simulink library "fft_library"  (Simulink 6.2)
values from neighbouring files (symbols this model uses):
  ActualCoeffs = exp(br_indices)    [butterfly_direct_mask.m]    (also in fft_stage_n_mask.m)
  MaxCoeffNum = 11    [biplex_core_mask.m]
  StepPeriod = FFTSize-FFTStage+max(0, FFTStage-MaxCoeffNum)    [fft_stage_n_mask.m]
  vlen = length(ActualCoeffs)    [fft_stage_n_mask.m]
undefined symbols (not defined in the file or in its folder): bit_reverse
libraries: xbsIndex_r3 x532, fft_library x29, delay_lib x9, reorder_library x7, twiddle_lib x1
(part 1 of 4)
settings Model: LastModifiedBy=hchen05

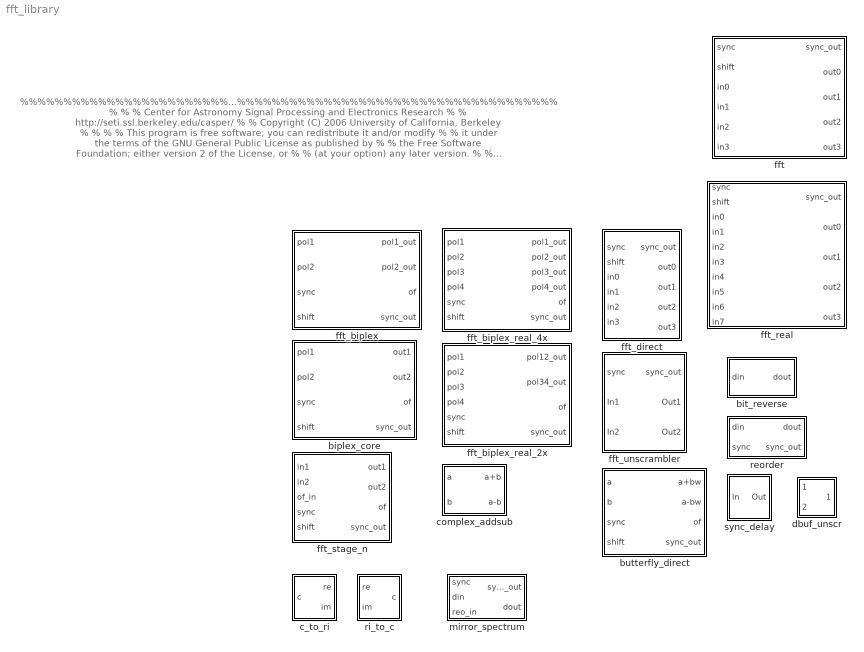
== system fft_library ==
  note: %%%%%%%%%%%%%%%%%%%%%%%%%%%%%%%%%%%%%%%%%%%%%%%%%%%%%%%%%%%%%%%%%%%%%%%%%%%%%%%
      | %                                                                             %
      | %   Center for Astronomy Signal Processing and Electronics Research           %
      | %   http://seti.ssl.berkeley.edu/casper/                                      %
      | %   Copyright (C) 2006 University of California, Berkeley                     %
      | %                                                                             %
      | %   This program is free software; you can redistribute it and/or modify      %
      | %   it under the terms of the GNU General Public License as published by      %
      | %   the Free Software Foundation; either version 2 of the License, or         %
      | %   (at your option) any later version.                                       %
      | %                                                                             %
      | %   This program is distributed in the hope that it will be useful,           %
      | %   but WITHOUT ANY WARRANTY; without even the implied warranty of            %
      | %   MERCHANTABILITY or FITNESS FOR A PARTICULAR PURPOSE.  See the             %
      | %   GNU General Public License for more details.                              %
      | %                                                                             %
      | %   You should have received a copy of the GNU General Public License along   %
      | %   with this program; if not, write to the Free Software Foundation, Inc.,   %
      | %   51 Franklin Street, Fifth Floor, Boston, MA 02110-1301 USA.               %
      | %                                                                             %
      | %%%%%%%%%%%%%%%%%%%%%%%%%%%%%%%%%%%%%%%%%%%%%%%%%%%%%%%%%%%%%%%%%%%%%%%%%%%%%%%
  biplex_core : Subsystem  mask{FFTSize=2, BitWidth=18, quantization=Truncate, overflow=Wrap, add_latency=2, mult_latency=3, bram_latency=2}
      mask prompts: FFTSize "Size of FFT: (2^? pnts)"; BitWidth "Bitwidth: (Max Efficiency at 18 bits)"; quantization "Quantization Behavior"; overflow "Overflow Behavior"; add_latency "Add Latency"; mult_latency "Mult Latency"; bram_latency "BRAM Latency"
      mask init:
      | biplex_core_mask;
      mask StyleString: edit,edit,popup(Truncate|Round  (unbiased: +/- Inf)|Round  (unbiased: Even Values)),popup(Wrap|Saturate|Error),edit,edit,edit
  bit_reverse : Subsystem  mask{n_bits=3}
      mask prompts: n_bits "Number of bits"
      mask init:
      | bit_reverse_mask;
      mask Display: fprintf('%d bits', n_bits)
  butterfly_direct : Subsystem  mask(butterfly_direct){FFTSize=5, Coeffs=0:3, StepPeriod=0, BitWidth=18, add_latency=4, mult_latency=4, bram_latency=4, use_bram=off, quantization=Round  (unbiased: Even Values), overflow=Wrap}
      mask prompts: FFTSize "Size of FFT: (2^?)"; Coeffs "Coefficients: (0 to 2^(FFTSize-1)-1)"; StepPeriod "Coefficient Step Period: (2^?)"; BitWidth "Output Bitwidth:"; add_latency "Add Latency"; mult_latency "Mult Latency"; bram_latency "BRAM Latency"; use_bram "Store Coefficients in BRAM"; quantization "Quantization Behavior"; overflow "Overflow Behavior"
      mask init:
      | butterfly_direct_mask;
      mask StyleString: edit,edit,edit,edit,edit,edit,edit,checkbox,popup(Truncate|Round  (unbiased: +/- Inf)|Round  (unbiased: Even Values)),popup(Wrap|Saturate|Error)
  c_to_ri : Subsystem  mask{BitWidth=18}
      mask prompts: BitWidth "Bit Width:"
  complex_addsub : Subsystem  mask{BitWidth=18, add_latency=2}
      mask prompts: BitWidth "Bit Wdith?"; add_latency "add latency?"
  dbuf_unscr : Subsystem  mask(dbuf_unscr){FFTSize=5, n_inputs=2, banknum=1, bram_latency=4}
      mask prompts: FFTSize "Size of FFT: (2^?)"; n_inputs "Number of Simultaneous Inputs: (2^?)"; banknum "Handling input #: (1 to # inputs)"; bram_latency "BRAM Latency"
      mask init:
      | biplex_len = FFTSize - n_inputs;
      | r = biplex_len - n_inputs;
  fft : Subsystem  mask{FFTSize=5, BitWidth=18, n_inputs=2, quantization=Round  (unbiased: Even Values), overflow=Wrap, add_latency=2, mult_latency=3, bram_latency=2}
      mask prompts: FFTSize "Size of FFT: (2^?)"; BitWidth "Bit Width"; n_inputs "Number of Simultaneous Inputs: (2^?)"; quantization "Quantization Behavior"; overflow "Overflow Behavior"; add_latency "Add Latency"; mult_latency "Mult Latency"; bram_latency "BRAM Latency"
      mask init:
      | fft_mask;
      mask StyleString: edit,edit,edit,popup(Truncate|Round  (unbiased: +/- Inf)|Round  (unbiased: Even Values)),popup(Wrap|Saturate|Error),edit,edit,edit
  fft_biplex : Subsystem  mask(fft_biplex){FFTSize=2, BitWidth=18, quantization=Truncate, overflow=Wrap, add_latency=2, mult_latency=3, bram_latency=2}
      mask prompts: FFTSize "Size of FFT: (2^? pnts)"; BitWidth "Bitwidth: (Max Efficiency at 18 bits)"; quantization "Quantization Behavior"; overflow "Overflow Behavior"; add_latency "Add Latency"; mult_latency "Mult Latency"; bram_latency "BRAM Latency"
      mask init:
      | cursys = gcb;
      | disp(cursys);
      | biplex_core = [cursys,'/biplex_core'];
      | if ~strcmp(get_param(biplex_core, 'quantization'), quantization),
      |     set_param(biplex_core, 'quantization', quantization);
      | end
      | if ~strcmp(get_param(biplex_core, 'overflow'), overflow),
      |     set_param(biplex_core, 'overflow', overflow);
      | end
      mask StyleString: edit,edit,popup(Truncate|Round  (unbiased: +/- Inf)|Round  (unbiased: Even Values)),popup(Wrap|Saturate|Error),edit,edit,edit
  fft_biplex_real_2x : Subsystem  mask{FFTSize=2, BitWidth=18, quantization=Round  (unbiased: Even Values), overflow=Wrap, add_latency=2, mult_latency=3, bram_latency=2}
      mask prompts: FFTSize "Size of FFT: (2^? pnts)"; BitWidth "Bitwidth: (Max Efficiency at 18 bits)"; quantization "Quantization Behavior"; overflow "Overflow Behavior"; add_latency "Add Latency"; mult_latency "Mult Latency"; bram_latency "BRAM Latency"
      mask init:
      | cursys = gcb;
      | disp(cursys);
      | biplex_core = [cursys,'/biplex_core'];
      | if ~strcmp(get_param(biplex_core, 'quantization'), quantization),
      |     set_param(biplex_core, 'quantization', quantization);
      | end
      mask StyleString: edit,edit,popup(Truncate|Round  (unbiased: +/- Inf)|Round  (unbiased: Even Values)),popup(Wrap|Saturate|Error),edit,edit,edit
  fft_biplex_real_4x : Subsystem  mask(fft_biplex_real_4x){FFTSize=4, BitWidth=18, quantization=Round  (unbiased: Even Values), overflow=Wrap, add_latency=2, mult_latency=3, bram_latency=2}
      mask prompts: FFTSize "Size of FFT: (2^? pnts)"; BitWidth "Bitwidth: (Max Efficiency at 18 bits)"; quantization "Quantization Behavior"; overflow "Overflow Behavior"; add_latency "Add Latency"; mult_latency "Mult Latency"; bram_latency "BRAM Latency"
      mask init:
      | cursys = gcb;
      | disp(cursys);
      | 
      | BRAMSize = 18432;
      | DelayBramThresh = 1/4;  % Use bram when delays will fill this fraction of a BRAM
      | 
      | biplex_core = [cursys,'/biplex_core'];
      | if ~strcmp(get_param(biplex_core, 'quantization'), quantization),
      |     set_param(biplex_core, 'quantization', quantization);
      | end
      | 
      | % Implement delays normally or in BRAM
      | 
      | if (2^(FFTSize-1) * 2*BitWidth >= DelayBramThresh*BRAMSize),
      |     delay_bram = 'on';
      | else,
      |     delay_bram = 'off';
      | end
      | 
      | delays = {'delay0', 'delay1'};
      | for i=1:length(delays),
      |     full_path = [cursys,'/bi_real_unscr_4x/',delays{i}];
      |     if 2^(FFTSize-1) > 16,
      |         delay_type = 'delay_bram';
      |     else,
      |         delay_type = 'delay_slr';
      |     end
      |     if ~strcmp(get_param(full_path, 'BlockChoice'), delay_type),
      |         set_param(full_path, 'BlockChoice', delay_type)
      |     end
      | end
      mask StyleString: edit,edit,popup(Truncate|Round  (unbiased: +/- Inf)|Round  (unbiased: Even Values)),popup(Wrap|Saturate|Error),edit,edit,edit
  fft_direct : Subsystem  mask{FFTSize=2, BitWidth=18, add_latency=2, mult_latency=3, bram_latency=2, quantization=Truncate, overflow=Wrap, MapTail=off, LargerFFTSize=5, StartStage=3}
      mask prompts: FFTSize "Size of FFT: (2^?)"; BitWidth "Bit Width"; add_latency "Add Latency"; mult_latency "Mult Latency"; bram_latency "BRAM Latency"; quantization "Quantization Behavior"; overflow "Overflow Behavior"; MapTail "Map Tail of Larger FFT"; LargerFFTSize "Size of Larger FFT (2^?):"; StartStage "Start Stage of Map Tail:"
      mask init:
      | fft_direct_mask;
      mask StyleString: edit,edit,edit,edit,edit,popup(Truncate|Round  (unbiased: +/- Inf)|Round  (unbiased: Even Values)),popup(Wrap|Saturate|Error),checkbox,edit,edit
      mask CallbackString:
      | |||||||if strcmp(get_param(gcb,'Maptail'),'on')
      |     set_param(gcb,'MaskVisibilities',{'on','on','on','on','on','on','on','on','on','on'});
      | else
      |     set_param(gcb,'MaskVisibilities',{'on','on','on','on','on','on','on','on','off','off'});
      | end||
  fft_real : Subsystem  mask{FFTSize=8, BitWidth=18, n_inputs=3, quantization=Round  (unbiased: Even Values), overflow=Wrap, add_latency=2, mult_latency=3, bram_latency=2}
      mask prompts: FFTSize "Size of FFT: (2^?)"; BitWidth "Bit Width"; n_inputs "Number of Simultaneous Inputs: (2^?)"; quantization "Quantization Behavior"; overflow "Overflow Behavior"; add_latency "Add Latency"; mult_latency "Mult Latency"; bram_latency "BRAM Latency"
      mask init:
      | fft_real_mask;
      mask StyleString: edit,edit,edit,popup(Truncate|Round  (unbiased: +/- Inf)|Round  (unbiased: Even Values)),popup(Wrap|Saturate|Error),edit,edit,edit
  fft_stage_n : Subsystem  mask(fft_stage){FFTSize=5, FFTStage=3, BitWidth=18, DelayBram=off, CoeffBram=off, MaxCoeffNum=12, quantization=Truncate, overflow=Wrap, add_latency=3, mult_latency=2, bram_latency=2}
      mask prompts: FFTSize "Size of FFT: (2^? pnts)"; FFTStage "Stage of FFT:"; BitWidth "Output Bitwidth:"; DelayBram "Implement Delays in BRAM:"; CoeffBram "Store Coefficients in BRAM:"; MaxCoeffNum "Maximum Coefficient Depth: (2^?)"; quantization "Quantization Behavior"; overflow "Overflow Behavior"; add_latency "Add Latency"; mult_latency "Mult Latency"; bram_latency "BRAM Latency"
      mask init:
      | fft_stage_n_mask;
      mask StyleString: edit,edit,edit,checkbox,checkbox,edit,popup(Truncate|Round  (unbiased: +/- Inf)|Round  (unbiased: Even Values)),popup(Wrap|Saturate|Error),edit,edit,edit
  fft_unscrambler : Subsystem  mask{FFTSize=6, n_inputs=1, bram_latency=2}
      mask prompts: FFTSize "Size of FFT: (2^?)"; n_inputs "Number of Simultaneous Inputs: (2^?)"; bram_latency "BRAM Latency"
      mask init:
      | fft_unscrambler_mask;
  mirror_spectrum : Subsystem  mask{FFTSize=4, n_bits=18, reorder_latency=2}
      mask prompts: FFTSize "FFT Size (2^?):"; n_bits "Bit Width"; reorder_latency "Reorder Latency"
  reorder : Subsystem  mask{n_bits=2, bit_reverse=off, ping_pong=off, bram_latency=2}
      mask prompts: n_bits "Length of Vector: (2^?)"; bit_reverse "Bit Reverse"; ping_pong "Backwards"; bram_latency "BRAM Latency"
      mask init:
      | cursys = gcb;
      | disp(cursys);
      | set_param([cursys,'/crazy_cnt'], 'bit_reverse', bit_reverse);
      | set_param([cursys,'/crazy_cnt'], 'ping_pong', ping_pong);
  ri_to_c : Subsystem  mask{likes_cookies=off}
      mask prompts: likes_cookies "I think cookies are delicious"
  sync_delay : Subsystem  mask{DelayLen=4}
      mask prompts: DelayLen "Delay Length:"
      mask init:
      | BitWidth = max(2, ceil(log2(DelayLen+1)));
      | UseCounter = 1;
      | if DelayLen == 0,
      | 	UseCounter = 0;
      | end
      mask Display: fprintf('Z^-%d', DelayLen)

== system fft_library/biplex_core ==
  pol1 : Inport  Port=1  LatchInput=off
  pol2 : Inport  Port=2  LatchInput=off
  sync : Inport  Port=3  LatchInput=off
  shift : Inport  Port=4  LatchInput=off
  fft_stage_1 : Subsystem  mask(fft_stage){FFTSize=FFTSize, FFTStage=1, BitWidth=BitWidth, DelayBram=off, CoeffBram=off, MaxCoeffNum=MaxCoeffNum, quantization=Truncate, overflow=Wrap, add_latency=add_latency, mult_latency=mult_latency, bram_latency=bram_latency}
      mask prompts: FFTSize "Size of FFT: (2^? pnts)"; FFTStage "Stage of FFT:"; BitWidth "Output Bitwidth:"; DelayBram "Implement Delays in BRAM:"; CoeffBram "Store Coefficients in BRAM:"; MaxCoeffNum "Maximum Coefficient Depth: (2^?)"; quantization "Quantization Behavior"; overflow "Overflow Behavior"; add_latency "Add Latency"; mult_latency "Mult Latency"; bram_latency "BRAM Latency"
      mask init:
      | fft_stage_n_mask;
      mask StyleString: edit,edit,edit,checkbox,checkbox,edit,popup(Truncate|Round  (unbiased: +/- Inf)|Round  (unbiased: Even Values)),popup(Wrap|Saturate|Error),edit,edit,edit
  fft_stage_2 : Subsystem  mask(fft_stage){FFTSize=FFTSize, FFTStage=2, BitWidth=BitWidth, DelayBram=off, CoeffBram=off, MaxCoeffNum=MaxCoeffNum, quantization=Truncate, overflow=Wrap, add_latency=add_latency, mult_latency=mult_latency, bram_latency=bram_latency}
      mask prompts: FFTSize "Size of FFT: (2^? pnts)"; FFTStage "Stage of FFT:"; BitWidth "Output Bitwidth:"; DelayBram "Implement Delays in BRAM:"; CoeffBram "Store Coefficients in BRAM:"; MaxCoeffNum "Maximum Coefficient Depth: (2^?)"; quantization "Quantization Behavior"; overflow "Overflow Behavior"; add_latency "Add Latency"; mult_latency "Mult Latency"; bram_latency "BRAM Latency"
      mask init:
      | fft_stage_n_mask;
      mask StyleString: edit,edit,edit,checkbox,checkbox,edit,popup(Truncate|Round  (unbiased: +/- Inf)|Round  (unbiased: Even Values)),popup(Wrap|Saturate|Error),edit,edit,edit
  out1 : Outport
  out2 : Outport  Port=2
  of : Outport  Port=3
  sync_out : Outport  Port=4
  wires:
  pol1/1 -> fft_stage_1/1(in1)
  pol2/1 -> fft_stage_1/2(in2)
  sync/1 -> fft_stage_1/3(sync)
  shift/1 -> fft_stage_1/4(shift), fft_stage_2/5(shift)
  fft_stage_1/1(out1) -> fft_stage_2/1(in1)
  fft_stage_1/2(out2) -> fft_stage_2/2(in2)
  fft_stage_1/3(of) -> fft_stage_2/3(of_in)
  fft_stage_1/4(sync_out) -> fft_stage_2/4(sync)
  fft_stage_2/1(out1) -> out1/1
  fft_stage_2/2(out2) -> out2/1
  fft_stage_2/3(of) -> of/1
  fft_stage_2/4(sync_out) -> sync_out/1

== system fft_library/bit_reverse ==
  din : Inport  Port=1  LatchInput=off
  Concat : xbsIndex_r3/Concat  num_inputs=3  explicit_period=off  period=1  dbl_ovrd=off
  slice0 : xbsIndex_r3/Slice  mode=Lower Bit Location + Width  nbits=1  bit1=0  base1=MSB of Input  bit0=0  base0=LSB of Input  boolean_output=off  explicit_period=off  period=1  dbl_ovrd=off
  slice1 : xbsIndex_r3/Slice  mode=Lower Bit Location + Width  nbits=1  bit1=0  base1=MSB of Input  bit0=1  base0=LSB of Input  boolean_output=off  explicit_period=off  period=1  dbl_ovrd=off
  slice2 : xbsIndex_r3/Slice  mode=Lower Bit Location + Width  nbits=1  bit1=0  base1=MSB of Input  bit0=2  base0=LSB of Input  boolean_output=off  explicit_period=off  period=1  dbl_ovrd=off
  dout : Outport
  wires:
  din/1 -> slice0/1, slice1/1, slice2/1
  slice0/1 -> Concat/1
  slice1/1 -> Concat/2
  slice2/1 -> Concat/3
  Concat/1 -> dout/1

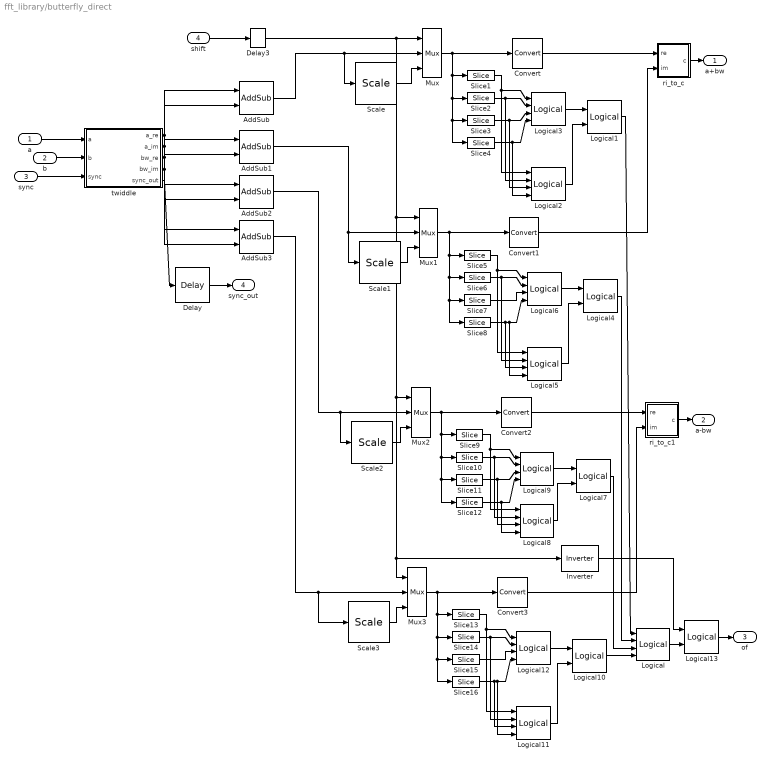
== system fft_library/butterfly_direct ==
  a : Inport  Port=1  LatchInput=off
  b : Inport  Port=2  LatchInput=off
  sync : Inport  Port=3  LatchInput=off
  shift : Inport  Port=4  LatchInput=off
  AddSub : xbsIndex_r3/AddSub  mode=Addition  precision=Full  arith_type=Unsigned  n_bits=8  bin_pt=2  quantization=Truncate  overflow=Wrap  latency=add_latency  explicit_period=off  period=1  use_carryin=off  use_carryout=off  en=off  dbl_ovrd=off  show_param=on  use_core=on  pipeline=on  use_rpm=on  gen_core=on
      settings: xl_area=[0, 0, 0, 0, 0, 0, 0]
  AddSub1 : xbsIndex_r3/AddSub  mode=Addition  precision=Full  arith_type=Unsigned  n_bits=8  bin_pt=2  quantization=Truncate  overflow=Wrap  latency=add_latency  explicit_period=off  period=1  use_carryin=off  use_carryout=off  en=off  dbl_ovrd=off  show_param=on  use_core=on  pipeline=on  use_rpm=on  gen_core=on
      settings: xl_area=[0, 0, 0, 0, 0, 0, 0]
  AddSub2 : xbsIndex_r3/AddSub  mode=Subtraction  precision=Full  arith_type=Unsigned  n_bits=8  bin_pt=2  quantization=Truncate  overflow=Wrap  latency=add_latency  explicit_period=off  period=1  use_carryin=off  use_carryout=off  en=off  dbl_ovrd=off  show_param=on  use_core=on  pipeline=on  use_rpm=on  gen_core=on
      settings: xl_area=[0, 0, 0, 0, 0, 0, 0]
  AddSub3 : xbsIndex_r3/AddSub  mode=Subtraction  precision=Full  arith_type=Unsigned  n_bits=8  bin_pt=2  quantization=Truncate  overflow=Wrap  latency=add_latency  explicit_period=off  period=1  use_carryin=off  use_carryout=off  en=off  dbl_ovrd=off  show_param=on  use_core=on  pipeline=on  use_rpm=on  gen_core=on
      settings: xl_area=[0, 0, 0, 0, 0, 0, 0]
  Convert{,1..3} (4 alike) : xbsIndex_r3/Convert  arith_type="Signed  (2's comp)"  n_bits=BitWidth  bin_pt=BitWidth-1  quantization="Round  (unbiased: Even Values)"  overflow=Wrap  latency=add_latency  explicit_period=off  period=1  dbl_ovrd=off  show_param=off  inserted_by_tool=off  pipeline=off
      settings: xl_area=[0, 0, 0, 0, 0, 0, 0]
  Delay : xbsIndex_r3/Delay  latency=2 * add_latency + 1  reg_retiming=off  explicit_period=off  period=1  en=off  accept_only_valid=off  init_zero=on  dbl_ovrd=off  show_param=off
      settings: xl_area=[0, 0, 0, 0, 0, 0, 0]
  Delay3 : xbsIndex_r3/Delay  latency=1  reg_retiming=off  explicit_period=off  period=1  en=off  accept_only_valid=off  init_zero=on  dbl_ovrd=off  show_param=off
      settings: xl_area=[0, 0, 0, 0, 0, 0, 0]
  Inverter : xbsIndex_r3/Inverter  latency=0  explicit_period=off  period=1  en=off  dbl_ovrd=off  show_param=off
      settings: xl_area=[0, 0, 0, 0, 0, 0, 0]
  Logical : xbsIndex_r3/Logical  logical_function=OR  inputs=4  precision=Full  arith_type=Unsigned  n_bits=8  bin_pt=2  align_bp=on  latency=1  explicit_period=off  period=1  en=off  dbl_ovrd=off  show_param=off
      settings: xl_area=[0, 0, 0, 0, 0, 0, 0]
  Logical{1,4,7,10} (4 alike) : xbsIndex_r3/Logical  logical_function=OR  inputs=2  precision=Full  arith_type=Unsigned  n_bits=8  bin_pt=2  align_bp=off  latency=1  explicit_period=off  period=1  en=off  dbl_ovrd=off  show_param=off
      settings: xl_area=[0, 0, 0, 0, 0, 0, 0]
  Logical{2,5,8,11} (4 alike) : xbsIndex_r3/Logical  logical_function=NOR  inputs=4  precision=Full  arith_type=Unsigned  n_bits=8  bin_pt=2  align_bp=off  latency=1  explicit_period=off  period=1  en=off  dbl_ovrd=off  show_param=off
      settings: xl_area=[0, 0, 0, 0, 0, 0, 0]
  Logical{3,6,9,12} (4 alike) : xbsIndex_r3/Logical  logical_function=AND  inputs=4  precision=Full  arith_type=Unsigned  n_bits=8  bin_pt=2  align_bp=off  latency=1  explicit_period=off  period=1  en=off  dbl_ovrd=off  show_param=off
      settings: xl_area=[0, 0, 0, 0, 0, 0, 0]
  Logical13 : xbsIndex_r3/Logical  logical_function=AND  inputs=2  precision=Full  arith_type=Unsigned  n_bits=8  bin_pt=2  align_bp=off  latency=1  explicit_period=off  period=1  en=off  dbl_ovrd=off  show_param=off
      settings: xl_area=[0, 0, 0, 0, 0, 0, 0]
  Mux{,1..3} (4 alike) : xbsIndex_r3/Mux  inputs=2  precision=Full  arith_type="Signed  (2's comp)"  n_bits=8  bin_pt=2  quantization=Truncate  overflow=Wrap  latency=1  explicit_period=off  period=1  en=off  dbl_ovrd=off  show_param=off  mux_type=off  use_rpm=off  gen_core=off
      settings: xl_area=[0, 0, 0, 0, 0, 0, 0]
  Scale{,1..3} (4 alike) : xbsIndex_r3/Scale  scale_factor=-1  explicit_period=off  period=1  dbl_ovrd=off
  Slice{1,5,9,13} (4 alike) : xbsIndex_r3/Slice  mode=Upper Bit Location + Width  nbits=1  bit1=0  base1=MSB of Input  bit0=0  base0=LSB of Input  boolean_output=on  explicit_period=off  period=1  dbl_ovrd=off
  Slice{2,6,10,14} (4 alike) : xbsIndex_r3/Slice  mode=Upper Bit Location + Width  nbits=1  bit1=-1  base1=MSB of Input  bit0=0  base0=LSB of Input  boolean_output=on  explicit_period=off  period=1  dbl_ovrd=off
  Slice{3,7,11,15} (4 alike) : xbsIndex_r3/Slice  mode=Upper Bit Location + Width  nbits=1  bit1=-2  base1=MSB of Input  bit0=0  base0=LSB of Input  boolean_output=on  explicit_period=off  period=1  dbl_ovrd=off
  Slice{4,8,12,16} (4 alike) : xbsIndex_r3/Slice  mode=Upper Bit Location + Width  nbits=1  bit1=-3  base1=MSB of Input  bit0=0  base0=LSB of Input  boolean_output=on  explicit_period=off  period=1  dbl_ovrd=off
  ri_to_c : Subsystem
  ri_to_c1 : Subsystem
  twiddle : Subsystem  BlockChoice=twiddle_general_3mult
      link override twiddle_coeff_0: BitWidth=BitWidth  add_latency=add_latency  mult_latency=mult_latency  bram_latency=bram_latency
      link override twiddle_coeff_1: BitWidth=BitWidth  add_latency=add_latency  mult_latency=mult_latency  bram_latency=bram_latency
      link override twiddle_general: Coeffs=ActualCoeffs  StepPeriod=StepPeriod  BitWidth=BitWidth  add_latency=add_latency  mult_latency=mult_latency  bram_latency=bram_latency
      link override twiddle_general/coeff_gen: BlockChoice=br_coeff_gen
      link override twiddle_general/coeff_gen/br_coeff_gen/ROM: distributed_mem=on
      link override twiddle_general/coeff_gen/br_coeff_gen/ROM1: distributed_mem=on
      link override twiddle_general/coeff_gen/static_coeff_gen/Constant: equ=P=C
      link override twiddle_general/coeff_gen/static_coeff_gen/Constant1: equ=P=C
      link override twiddle_general_3mult: Coeffs=ActualCoeffs  StepPeriod=StepPeriod  BitWidth=BitWidth  add_latency=add_latency  mult_latency=mult_latency  bram_latency=bram_latency
      link override twiddle_general_3mult/coeff_gen: BlockChoice=br_coeff_gen
      link override twiddle_general_4mult: Coeffs=Coeffs  StepPeriod=StepPeriod  BitWidth=BitWidth  add_latency=add_latency  mult_latency=mult_latency  bram_latency=bram_latency
      link override twiddle_stage_2: FFTSize=FFTSize  BitWidth=BitWidth  add_latency=add_latency  mult_latency=mult_latency  bram_latency=bram_latency
      settings: AttributesFormatString=%<BlockChoice>  TemplateBlock=twiddle_lib/twiddle  MemberBlocks=twiddle_coeff_0,twiddle_coeff_1,twiddle_general_3mult,twiddle_general_4mult,twiddle_stage_2
  a+bw : Outport
  a-bw : Outport  Port=2
  of : Outport  Port=3
  sync_out : Outport  Port=4
  wires:
  twiddle/5(sync_out) -> Delay/1
  twiddle/4(bw_im) -> AddSub3/2, AddSub1/2
  twiddle/3(bw_re) -> AddSub2/2, AddSub/2
  twiddle/2(a_im) -> AddSub3/1, AddSub1/1
  twiddle/1(a_re) -> AddSub2/1, AddSub/1
  sync/1 -> twiddle/3(sync)
  b/1 -> twiddle/2(b)
  a/1 -> twiddle/1(a)
  ri_to_c/1(c) -> a+bw/1
  ri_to_c1/1(c) -> a-bw/1
  Delay/1 -> sync_out/1
  AddSub/1 -> Mux/2, Scale/1
  AddSub1/1 -> Mux1/2, Scale1/1
  shift/1 -> Delay3/1
  Mux/1 -> Convert/1, Slice1/1, Slice2/1, Slice3/1, Slice4/1
  Scale/1 -> Mux/3
  Convert/1 -> ri_to_c/1(re)
  Slice1/1 -> Logical3/1, Logical2/1
  Slice2/1 -> Logical3/2, Logical2/2
  Slice3/1 -> Logical3/3, Logical2/3
  Slice4/1 -> Logical3/4, Logical2/4
  Logical3/1 -> Logical1/1
  Logical2/1 -> Logical1/2
  Logical1/1 -> Logical/1
  Mux1/1 -> Convert1/1, Slice5/1, Slice6/1, Slice7/1, Slice8/1
  Scale1/1 -> Mux1/3
  Convert1/1 -> ri_to_c/2(im)
  Slice5/1 -> Logical6/1, Logical5/1
  Slice6/1 -> Logical6/2, Logical5/2
  Slice7/1 -> Logical6/3
  Slice8/1 -> Logical6/4, Logical5/4, Logical5/3
  Logical6/1 -> Logical4/1
  Logical5/1 -> Logical4/2
  Logical4/1 -> Logical/2
  Mux2/1 -> Convert2/1, Slice9/1, Slice10/1, Slice11/1, Slice12/1
  Scale2/1 -> Mux2/3
  Convert2/1 -> ri_to_c1/1(re)
  Slice9/1 -> Logical9/1, Logical8/1
  Slice10/1 -> Logical9/2, Logical8/2
  Slice11/1 -> Logical9/3, Logical8/3
  Slice12/1 -> Logical9/4, Logical8/4
  Logical9/1 -> Logical7/1
  Logical8/1 -> Logical7/2
  AddSub2/1 -> Mux2/2, Scale2/1
  Mux3/1 -> Convert3/1, Slice13/1, Slice14/1, Slice15/1, Slice16/1
  Scale3/1 -> Mux3/3
  Convert3/1 -> ri_to_c1/2(im)
  Slice13/1 -> Logical12/1, Logical11/1
  Slice14/1 -> Logical12/2, Logical11/2
  Slice15/1 -> Logical12/3
  Slice16/1 -> Logical12/4, Logical11/4, Logical11/3
  Logical12/1 -> Logical10/1
  Logical11/1 -> Logical10/2
  Logical10/1 -> Logical/4
  AddSub3/1 -> Mux3/2, Scale3/1
  Logical7/1 -> Logical/3
  Delay3/1 -> Mux/1, Mux1/1, Mux2/1, Mux3/1, Inverter/1
  Logical/1 -> Logical13/2
  Logical13/1 -> of/1
  Inverter/1 -> Logical13/1

== system fft_library/c_to_ri ==
  c : Inport  Port=1  LatchInput=off
  Reinterpret : xbsIndex_r3/Reinterpret  force_arith_type=on  arith_type="Signed  (2's comp)"  force_bin_pt=on  bin_pt=BitWidth - 1  force_valid=on
  Reinterpret1 : xbsIndex_r3/Reinterpret  force_arith_type=on  arith_type="Signed  (2's comp)"  force_bin_pt=on  bin_pt=BitWidth - 1  force_valid=on
  Slice : xbsIndex_r3/Slice  mode=Upper Bit Location + Width  nbits=BitWidth  bit1=0  base1=MSB of Input  bit0=0  base0=LSB of Input  boolean_output=off  explicit_period=off  period=1  dbl_ovrd=off
  Slice1 : xbsIndex_r3/Slice  mode=Lower Bit Location + Width  nbits=BitWidth  bit1=0  base1=MSB of Input  bit0=0  base0=LSB of Input  boolean_output=off  explicit_period=off  period=1  dbl_ovrd=off
  re : Outport
  im : Outport  Port=2
  wires:
  Slice/1 -> Reinterpret/1
  Slice1/1 -> Reinterpret1/1
  Reinterpret/1 -> re/1
  Reinterpret1/1 -> im/1
  c/1 -> Slice/1, Slice1/1

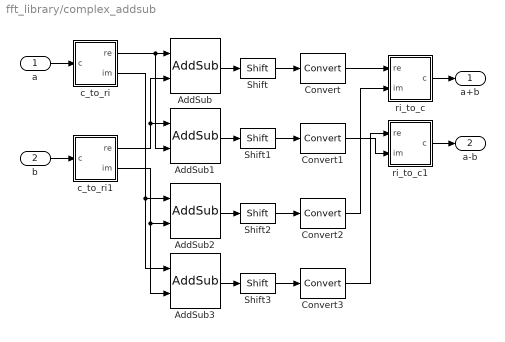
== system fft_library/complex_addsub ==
  a : Inport  Port=1  LatchInput=off
  b : Inport  Port=2  LatchInput=off
  AddSub : xbsIndex_r3/AddSub  mode=Addition  precision=Full  arith_type=Unsigned  n_bits=8  bin_pt=2  quantization=Truncate  overflow=Wrap  latency=add_latency  explicit_period=off  period=1  use_carryin=off  use_carryout=off  en=off  dbl_ovrd=off  show_param=off  use_core=on  pipeline=off  use_rpm=on  gen_core=off
      settings: xl_area=[0, 0, 0, 0, 0, 0, 0]
  AddSub1 : xbsIndex_r3/AddSub  mode=Subtraction  precision=Full  arith_type=Unsigned  n_bits=8  bin_pt=2  quantization=Truncate  overflow=Wrap  latency=add_latency  explicit_period=off  period=1  use_carryin=off  use_carryout=off  en=off  dbl_ovrd=off  show_param=off  use_core=on  pipeline=off  use_rpm=on  gen_core=off
      settings: xl_area=[0, 0, 0, 0, 0, 0, 0]
  AddSub2 : xbsIndex_r3/AddSub  mode=Subtraction  precision=Full  arith_type=Unsigned  n_bits=8  bin_pt=2  quantization=Truncate  overflow=Wrap  latency=add_latency  explicit_period=off  period=1  use_carryin=off  use_carryout=off  en=off  dbl_ovrd=off  show_param=off  use_core=on  pipeline=off  use_rpm=on  gen_core=off
      settings: xl_area=[0, 0, 0, 0, 0, 0, 0]
  AddSub3 : xbsIndex_r3/AddSub  mode=Addition  precision=Full  arith_type=Unsigned  n_bits=8  bin_pt=2  quantization=Truncate  overflow=Wrap  latency=add_latency  explicit_period=off  period=1  use_carryin=off  use_carryout=off  en=off  dbl_ovrd=off  show_param=off  use_core=on  pipeline=off  use_rpm=on  gen_core=off
      settings: xl_area=[0, 0, 0, 0, 0, 0, 0]
  Convert{,1..3} (4 alike) : xbsIndex_r3/Convert  arith_type="Signed  (2's comp)"  n_bits=BitWidth  bin_pt=BitWidth - 1  quantization="Round  (unbiased: Even Values)"  overflow=Wrap  latency=add_latency  explicit_period=off  period=1  dbl_ovrd=off  show_param=off  inserted_by_tool=off  pipeline=off
      settings: xl_area=[0, 0, 0, 0, 0, 0, 0]
  Shift{,1..3} (4 alike) : xbsIndex_r3/Shift  shift_dir=Right  shift_bits=1  precision=Full  arith_type="Signed  (2's comp)"  n_bits=8  bin_pt=2  quantization=Truncate  overflow=Wrap  latency=0  explicit_period=off  period=1  en=off  dbl_ovrd=off  show_param=off
      settings: xl_area=[0, 0, 0, 0, 0, 0, 0]
  c_to_ri : Subsystem
  c_to_ri1 : Subsystem
  ri_to_c : Subsystem
  ri_to_c1 : Subsystem
  a+b : Outport
  a-b : Outport  Port=2
  wires:
  Convert3/1 -> ri_to_c1/1(re)
  Convert1/1 -> ri_to_c1/2(im)
  AddSub/1 -> Shift/1
  AddSub1/1 -> Shift1/1
  AddSub2/1 -> Shift2/1
  AddSub3/1 -> Shift3/1
  c_to_ri/1(re) -> AddSub1/2, AddSub/1
  c_to_ri/2(im) -> AddSub2/1, AddSub3/1
  c_to_ri1/1(re) -> AddSub1/1, AddSub/2
  c_to_ri1/2(im) -> AddSub2/2, AddSub3/2
  Convert/1 -> ri_to_c/1(re)
  Convert2/1 -> ri_to_c/2(im)
  a/1 -> c_to_ri/1(c)
  ri_to_c/1(c) -> a+b/1
  ri_to_c1/1(c) -> a-b/1
  b/1 -> c_to_ri1/1(c)
  Shift/1 -> Convert/1
  Shift1/1 -> Convert1/1
  Shift2/1 -> Convert2/1
  Shift3/1 -> Convert3/1

== system fft_library/dbuf_unscr ==
  din : Inport  Port=1  LatchInput=off
  rst : Inport  Port=2  LatchInput=off
  Convert : xbsIndex_r3/Convert  arith_type=Boolean  n_bits=8  bin_pt=6  quantization=Truncate  overflow=Wrap  latency=0  explicit_period=off  period=1  dbl_ovrd=off  show_param=off  inserted_by_tool=off  pipeline=off
      settings: xl_area=[0, 0, 0, 0, 0, 0, 0]
  Delay : xbsIndex_r3/Delay  latency=bram_latency  reg_retiming=off  explicit_period=off  period=1  en=off  accept_only_valid=off  init_zero=on  dbl_ovrd=off  show_param=off
      settings: xl_area=[0, 0, 0, 0, 0, 0, 0]
  Delay1 : xbsIndex_r3/Delay  latency=1  reg_retiming=off  explicit_period=off  period=1  en=off  accept_only_valid=off  init_zero=on  dbl_ovrd=off  show_param=off
      settings: xl_area=[0, 0, 0, 0, 0, 0, 0]
  Inverter : xbsIndex_r3/Inverter  latency=0  explicit_period=off  period=1  en=off  dbl_ovrd=off  show_param=off
      settings: xl_area=[0, 0, 0, 0, 0, 0, 0]
  Mux : xbsIndex_r3/Mux  inputs=2  precision=Full  arith_type="Signed  (2's comp)"  n_bits=8  bin_pt=2  quantization=Truncate  overflow=Wrap  latency=1  explicit_period=off  period=1  en=off  dbl_ovrd=off  show_param=off  mux_type=off  use_rpm=off  gen_core=off
      settings: xl_area=[0, 0, 0, 0, 0, 0, 0]
  Single Port RAM : xbsIndex_r3/Single Port RAM  depth=2^biplex_len  initVector=0  write_mode=Read Before Write  latency=bram_latency  init_zero=on  explicit_period=off  period=1  rst=off  init_reg=0  en=off  dbl_ovrd=off  show_param=off  distributed_mem=off  use_rpm=off  gen_core=off
      settings: xl_area=[0, 0, 0, 0, 0, 0, 0]
  Single Port RAM1 : xbsIndex_r3/Single Port RAM  depth=2^biplex_len  initVector=0  write_mode=Read Before Write  latency=bram_latency  init_zero=on  explicit_period=off  period=1  rst=off  init_reg=0  en=off  dbl_ovrd=off  show_param=off  distributed_mem=off  use_rpm=off  gen_core=off
      settings: xl_area=[0, 0, 0, 0, 0, 0, 0]
  unscramble_cnt : Subsystem
  dout : Outport
  wires:
  unscramble_cnt/2(bank1_addr) -> Single Port RAM/1
  Delay/1 -> Mux/1
  unscramble_cnt/1(mode) -> Delay/1, Convert/1
  unscramble_cnt/3(bank2_addr) -> Single Port RAM1/1
  Mux/1 -> dout/1
  rst/1 -> unscramble_cnt/1(rst)
  din/1 -> Delay1/1
  Delay1/1 -> Single Port RAM/2, Single Port RAM1/2
  Convert/1 -> Inverter/1, Single Port RAM1/3
  Single Port RAM1/1 -> Mux/2
  Single Port RAM/1 -> Mux/3
  Inverter/1 -> Single Port RAM/3

== system fft_library/fft ==
  sync : Inport  Port=1  LatchInput=off
  shift : Inport  Port=2  LatchInput=off
  in0 : Inport  Port=3  LatchInput=off
  in1 : Inport  Port=4  LatchInput=off
  in2 : Inport  Port=5  LatchInput=off
  in3 : Inport  Port=6  LatchInput=off
  fft_biplex0 : fft_library/fft_biplex  FFTSize=FFTSize-n_inputs  BitWidth=BitWidth  quantization="Round  (unbiased: Even Values)"  overflow=Wrap  add_latency=add_latency  mult_latency=mult_latency  bram_latency=bram_latency
  fft_biplex1 : fft_library/fft_biplex  FFTSize=FFTSize-n_inputs  BitWidth=BitWidth  quantization="Round  (unbiased: Even Values)"  overflow=Wrap  add_latency=add_latency  mult_latency=mult_latency  bram_latency=bram_latency
  fft_direct : fft_library/fft_direct  FFTSize=n_inputs  BitWidth=BitWidth  add_latency=add_latency  mult_latency=mult_latency  bram_latency=bram_latency  quantization="Round  (unbiased: Even Values)"  overflow=Wrap  MapTail=on  LargerFFTSize=FFTSize  StartStage=FFTSize-n_inputs+1
  fft_unscrambler : fft_library/fft_unscrambler  FFTSize=FFTSize  n_inputs=n_inputs  bram_latency=bram_latency
  slice : xbsIndex_r3/Slice  mode=Lower Bit Location + Width  nbits=n_inputs  bit1=0  base1=MSB of Input  bit0=FFTSize-n_inputs  base0=LSB of Input  boolean_output=off  explicit_period=off  period=1  dbl_ovrd=off
  sync_out : Outport
  out0 : Outport  Port=2
  out1 : Outport  Port=3
  out2 : Outport  Port=4
  out3 : Outport  Port=5
  wires:
  in0/1 -> fft_biplex0/1
  in1/1 -> fft_biplex0/2
  shift/1 -> fft_biplex0/4, fft_biplex1/4, slice/1
  sync/1 -> fft_biplex0/3, fft_biplex1/3
  in2/1 -> fft_biplex1/1
  in3/1 -> fft_biplex1/2
  slice/1 -> fft_direct/2
  fft_biplex0/4 -> fft_direct/1
  fft_biplex0/1 -> fft_direct/3
  fft_biplex0/2 -> fft_direct/4
  fft_biplex1/1 -> fft_direct/5
  fft_biplex1/2 -> fft_direct/6
  fft_direct/1 -> fft_unscrambler/1
  fft_unscrambler/1 -> sync_out/1
  fft_direct/2 -> fft_unscrambler/2
  fft_unscrambler/2 -> out0/1
  fft_direct/3 -> fft_unscrambler/3
  fft_unscrambler/3 -> out1/1
  fft_direct/4 -> fft_unscrambler/4
  fft_unscrambler/4 -> out2/1
  fft_direct/5 -> fft_unscrambler/5
  fft_unscrambler/5 -> out3/1

== system fft_library/fft_biplex ==
  pol1 : Inport  Port=1  LatchInput=off
  pol2 : Inport  Port=2  LatchInput=off
  sync : Inport  Port=3  LatchInput=off
  shift : Inport  Port=4  LatchInput=off
  biplex_core : fft_library/biplex_core  FFTSize=FFTSize  BitWidth=BitWidth  quantization=Truncate  overflow=Wrap  add_latency=add_latency  mult_latency=mult_latency  bram_latency=bram_latency
  biplex_cplx_unscrambler : Subsystem
  pol1_out : Outport
  pol2_out : Outport  Port=2
  of : Outport  Port=3
  sync_out : Outport  Port=4
  wires:
  pol1/1 -> biplex_core/1
  pol2/1 -> biplex_core/2
  sync/1 -> biplex_core/3
  shift/1 -> biplex_core/4
  biplex_cplx_unscrambler/1(pol1) -> pol1_out/1
  biplex_cplx_unscrambler/2(pol2) -> pol2_out/1
  biplex_cplx_unscrambler/3(sync_out) -> sync_out/1
  biplex_core/3 -> of/1
  biplex_core/1 -> biplex_cplx_unscrambler/1(even)
  biplex_core/2 -> biplex_cplx_unscrambler/2(odd)
  biplex_core/4 -> biplex_cplx_unscrambler/3(sync)

== system fft_library/fft_biplex_real_2x ==
  pol1 : Inport  Port=1  LatchInput=off
  pol2 : Inport  Port=2  LatchInput=off
  pol3 : Inport  Port=3  LatchInput=off
  pol4 : Inport  Port=4  LatchInput=off
  sync : Inport  Port=5  LatchInput=off
  shift : Inport  Port=6  LatchInput=off
  bi_real_unscr_2x : Subsystem  mask{FFTSize=FFTSize, n_bits=BitWidth, add_latency=add_latency, bram_latency=bram_latency}
      mask prompts: FFTSize "Size of FFT (2^?):"; n_bits "Sample Bit Width"; add_latency "Add Latency"; bram_latency "BRAM Latency"
  biplex_core : fft_library/biplex_core  FFTSize=FFTSize  BitWidth=BitWidth  quantization="Round  (unbiased: Even Values)"  overflow=Wrap  add_latency=add_latency  mult_latency=mult_latency  bram_latency=bram_latency
  ri_to_c : Subsystem
  ri_to_c1 : Subsystem
  pol12_out : Outport
  pol34_out : Outport  Port=2
  of : Outport  Port=3
  sync_out : Outport  Port=4
  wires:
  bi_real_unscr_2x/3(sync_out) -> sync_out/1
  bi_real_unscr_2x/2(pol34_out) -> pol34_out/1
  bi_real_unscr_2x/1(pol12_out) -> pol12_out/1
  shift/1 -> biplex_core/4
  sync/1 -> biplex_core/3
  pol4/1 -> ri_to_c1/2(im)
  ri_to_c1/1(c) -> biplex_core/2
  pol3/1 -> ri_to_c1/1(re)
  pol2/1 -> ri_to_c/2(im)
  ri_to_c/1(c) -> biplex_core/1
  pol1/1 -> ri_to_c/1(re)
  biplex_core/3 -> of/1
  biplex_core/1 -> bi_real_unscr_2x/1(even)
  biplex_core/2 -> bi_real_unscr_2x/2(odd)
  biplex_core/4 -> bi_real_unscr_2x/3(sync)

== system fft_library/fft_biplex_real_4x ==
  pol1 : Inport  Port=1  LatchInput=off
  pol2 : Inport  Port=2  LatchInput=off
  pol3 : Inport  Port=3  LatchInput=off
  pol4 : Inport  Port=4  LatchInput=off
  sync : Inport  Port=5  LatchInput=off
  shift : Inport  Port=6  LatchInput=off
  bi_real_unscr_4x : Subsystem
  biplex_core : fft_library/biplex_core  FFTSize=FFTSize  BitWidth=BitWidth  quantization="Round  (unbiased: Even Values)"  overflow=Wrap  add_latency=add_latency  mult_latency=mult_latency  bram_latency=bram_latency
  ri_to_c : Subsystem
  ri_to_c1 : Subsystem
  pol1_out : Outport
  pol2_out : Outport  Port=2
  pol3_out : Outport  Port=3
  pol4_out : Outport  Port=4
  of : Outport  Port=5
  sync_out : Outport  Port=6
  wires:
  biplex_core/4 -> bi_real_unscr_4x/3(sync)
  biplex_core/2 -> bi_real_unscr_4x/2(odd)
  biplex_core/1 -> bi_real_unscr_4x/1(even)
  biplex_core/3 -> of/1
  pol1/1 -> ri_to_c/1(re)
  ri_to_c/1(c) -> biplex_core/1
  pol2/1 -> ri_to_c/2(im)
  pol3/1 -> ri_to_c1/1(re)
  ri_to_c1/1(c) -> biplex_core/2
  pol4/1 -> ri_to_c1/2(im)
  sync/1 -> biplex_core/3
  shift/1 -> biplex_core/4
  bi_real_unscr_4x/1(pol1_out) -> pol1_out/1
  bi_real_unscr_4x/2(pol2_out) -> pol2_out/1
  bi_real_unscr_4x/3(pol3_out) -> pol3_out/1
  bi_real_unscr_4x/4(pol4_out) -> pol4_out/1
  bi_real_unscr_4x/5(sync_out) -> sync_out/1

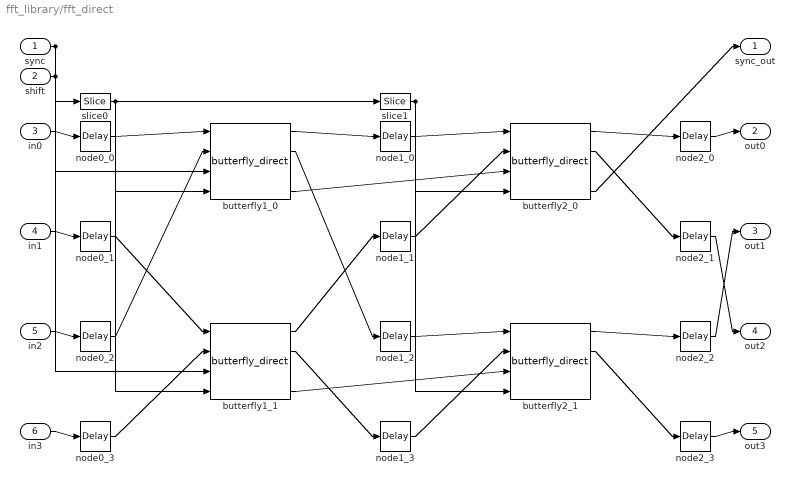
== system fft_library/fft_direct ==
  sync : Inport  Port=1  LatchInput=off
  shift : Inport  Port=2  LatchInput=off
  in0 : Inport  Port=3  LatchInput=off
  in1 : Inport  Port=4  LatchInput=off
  in2 : Inport  Port=5  LatchInput=off
  in3 : Inport  Port=6  LatchInput=off
  butterfly1_0 : fft_library/butterfly_direct  FFTSize=2  Coeffs=[0]  StepPeriod=0  BitWidth=BitWidth  add_latency=add_latency  mult_latency=mult_latency  bram_latency=bram_latency  use_bram=off  quantization=Truncate  overflow=Wrap
  butterfly1_1 : fft_library/butterfly_direct  FFTSize=2  Coeffs=[0]  StepPeriod=0  BitWidth=BitWidth  add_latency=add_latency  mult_latency=mult_latency  bram_latency=bram_latency  use_bram=off  quantization=Truncate  overflow=Wrap
  butterfly2_0 : fft_library/butterfly_direct  FFTSize=2  Coeffs=[0]  StepPeriod=0  BitWidth=BitWidth  add_latency=add_latency  mult_latency=mult_latency  bram_latency=bram_latency  use_bram=off  quantization=Truncate  overflow=Wrap
  butterfly2_1 : fft_library/butterfly_direct  FFTSize=2  Coeffs=[1]  StepPeriod=0  BitWidth=BitWidth  add_latency=add_latency  mult_latency=mult_latency  bram_latency=bram_latency  use_bram=off  quantization=Truncate  overflow=Wrap
  node0_{0..3} (4 alike) : xbsIndex_r3/Delay  latency=0  reg_retiming=off  explicit_period=off  period=1  en=off  accept_only_valid=off  init_zero=on  dbl_ovrd=off  show_param=off
      settings: xl_area=[0, 0, 0, 0, 0, 0, 0]
  node1_{0..3} (4 alike) : xbsIndex_r3/Delay  latency=0  reg_retiming=off  explicit_period=off  period=1  en=off  accept_only_valid=off  init_zero=on  dbl_ovrd=off  show_param=off
      settings: xl_area=[0, 0, 0, 0, 0, 0, 0]
  node2_{0..3} (4 alike) : xbsIndex_r3/Delay  latency=0  reg_retiming=off  explicit_period=off  period=1  en=off  accept_only_valid=off  init_zero=on  dbl_ovrd=off  show_param=off
      settings: xl_area=[0, 0, 0, 0, 0, 0, 0]
  slice0 : xbsIndex_r3/Slice  mode=Lower Bit Location + Width  nbits=1  bit1=0  base1=MSB of Input  bit0=0  base0=LSB of Input  boolean_output=on  explicit_period=off  period=1  dbl_ovrd=off
  slice1 : xbsIndex_r3/Slice  mode=Lower Bit Location + Width  nbits=1  bit1=0  base1=MSB of Input  bit0=1  base0=LSB of Input  boolean_output=on  explicit_period=off  period=1  dbl_ovrd=off
  sync_out : Outport
  out0 : Outport  Port=2
  out1 : Outport  Port=3
  out2 : Outport  Port=4
  out3 : Outport  Port=5
  wires:
  in0/1 -> node0_0/1
  in1/1 -> node0_1/1
  in2/1 -> node0_2/1
  in3/1 -> node0_3/1
  shift/1 -> slice0/1, slice1/1
  node2_0/1 -> out0/1
  node2_1/1 -> out2/1
  node2_2/1 -> out1/1
  node2_3/1 -> out3/1
  node0_0/1 -> butterfly1_0/1
  node0_2/1 -> butterfly1_0/2
  butterfly1_0/1 -> node1_0/1
  butterfly1_0/2 -> node1_2/1
  sync/1 -> butterfly1_0/3, butterfly1_1/3
  slice0/1 -> butterfly1_0/4, butterfly1_1/4
  node0_1/1 -> butterfly1_1/1
  node0_3/1 -> butterfly1_1/2
  butterfly1_1/1 -> node1_1/1
  butterfly1_1/2 -> node1_3/1
  node1_0/1 -> butterfly2_0/1
  node1_1/1 -> butterfly2_0/2
  butterfly2_0/1 -> node2_0/1
  butterfly2_0/2 -> node2_1/1
  butterfly1_0/4 -> butterfly2_0/3
  butterfly2_0/4 -> sync_out/1
  slice1/1 -> butterfly2_0/4, butterfly2_1/4
  node1_2/1 -> butterfly2_1/1
  node1_3/1 -> butterfly2_1/2
  butterfly2_1/1 -> node2_2/1
  butterfly2_1/2 -> node2_3/1
  butterfly1_1/4 -> butterfly2_1/3

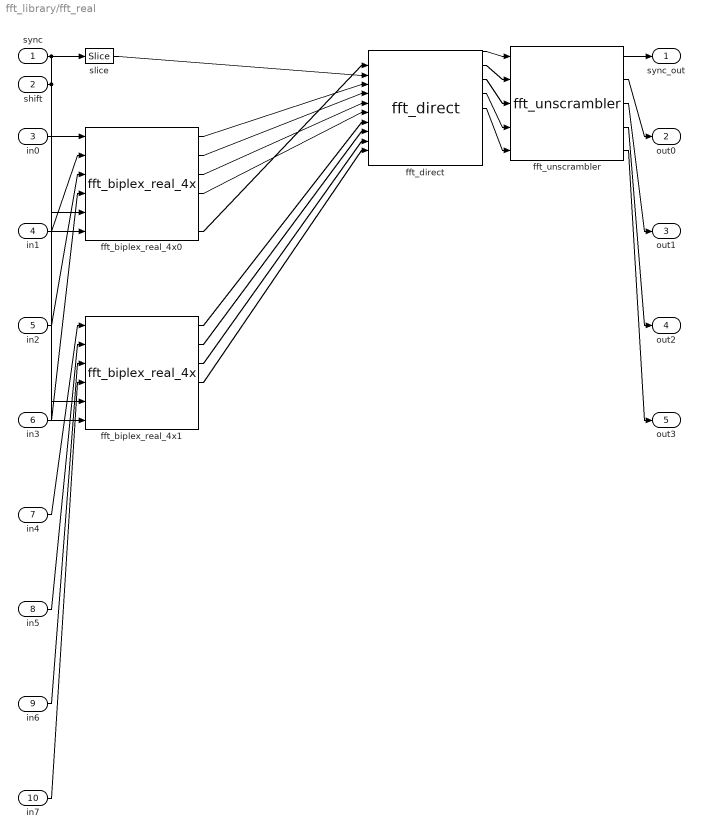
== system fft_library/fft_real ==
  sync : Inport  Port=1  LatchInput=off
  shift : Inport  Port=2  LatchInput=off
  in0 : Inport  Port=3  LatchInput=off
  in1 : Inport  Port=4  LatchInput=off
  in2 : Inport  Port=5  LatchInput=off
  in3 : Inport  Port=6  LatchInput=off
  in4 : Inport  Port=7  LatchInput=off
  in5 : Inport  Port=8  LatchInput=off
  in6 : Inport  Port=9  LatchInput=off
  in7 : Inport  Port=10  LatchInput=off
  fft_biplex_real_4x0 : fft_library/fft_biplex_real_4x  FFTSize=FFTSize-n_inputs  BitWidth=BitWidth  quantization="Round  (unbiased: Even Values)"  overflow=Wrap  add_latency=add_latency  mult_latency=mult_latency  bram_latency=bram_latency
  fft_biplex_real_4x1 : fft_library/fft_biplex_real_4x  FFTSize=FFTSize-n_inputs  BitWidth=BitWidth  quantization="Round  (unbiased: Even Values)"  overflow=Wrap  add_latency=add_latency  mult_latency=mult_latency  bram_latency=bram_latency
  fft_direct : fft_library/fft_direct  FFTSize=n_inputs  BitWidth=BitWidth  add_latency=add_latency  mult_latency=mult_latency  bram_latency=bram_latency  quantization="Round  (unbiased: Even Values)"  overflow=Wrap  MapTail=on  LargerFFTSize=FFTSize  StartStage=FFTSize-n_inputs+1
  fft_unscrambler : fft_library/fft_unscrambler  FFTSize=FFTSize-1  n_inputs=n_inputs-1  bram_latency=bram_latency
  slice : xbsIndex_r3/Slice  mode=Lower Bit Location + Width  nbits=n_inputs  bit1=0  base1=MSB of Input  bit0=FFTSize-n_inputs  base0=LSB of Input  boolean_output=off  explicit_period=off  period=1  dbl_ovrd=off
  sync_out : Outport
  out0 : Outport  Port=2
  out1 : Outport  Port=3
  out2 : Outport  Port=4
  out3 : Outport  Port=5
  wires:
  in0/1 -> fft_biplex_real_4x0/1
  in1/1 -> fft_biplex_real_4x0/2
  in2/1 -> fft_biplex_real_4x0/3
  in3/1 -> fft_biplex_real_4x0/4
  shift/1 -> fft_biplex_real_4x0/6, fft_biplex_real_4x1/6, slice/1
  sync/1 -> fft_biplex_real_4x0/5, fft_biplex_real_4x1/5
  in4/1 -> fft_biplex_real_4x1/1
  in5/1 -> fft_biplex_real_4x1/2
  in6/1 -> fft_biplex_real_4x1/3
  in7/1 -> fft_biplex_real_4x1/4
  slice/1 -> fft_direct/2
  fft_biplex_real_4x0/6 -> fft_direct/1
  fft_biplex_real_4x0/1 -> fft_direct/3
  fft_biplex_real_4x0/2 -> fft_direct/4
  fft_biplex_real_4x0/3 -> fft_direct/5
  fft_biplex_real_4x0/4 -> fft_direct/6
  fft_biplex_real_4x1/1 -> fft_direct/7
  fft_biplex_real_4x1/2 -> fft_direct/8
  fft_biplex_real_4x1/3 -> fft_direct/9
  fft_biplex_real_4x1/4 -> fft_direct/10
  fft_direct/1 -> fft_unscrambler/1
  fft_unscrambler/1 -> sync_out/1
  fft_direct/2 -> fft_unscrambler/2
  fft_unscrambler/2 -> out0/1
  fft_direct/3 -> fft_unscrambler/3
  fft_unscrambler/3 -> out1/1
  fft_direct/4 -> fft_unscrambler/4
  fft_unscrambler/4 -> out2/1
  fft_direct/5 -> fft_unscrambler/5
  fft_unscrambler/5 -> out3/1

== system fft_library/fft_stage_n ==
  in1 : Inport  Port=1  LatchInput=off
  in2 : Inport  Port=2  LatchInput=off
  of_in : Inport  Port=3  LatchInput=off
  sync : Inport  Port=4  LatchInput=off
  shift : Inport  Port=5  LatchInput=off
  Counter : xbsIndex_r3/Counter  cnt_type=Free Running  n_bits=FFTSize-FFTStage+1  bin_pt=0  arith_type=Unsigned  start_count=0  cnt_to=Inf  cnt_by_val=1  operation=Up  explicit_period=off  period=1  load_pin=off  rst=on  en=off  dbl_ovrd=off  show_param=off  use_rpm=off  gen_core=on
      settings: xl_area=[0, 0, 0, 0, 0, 0, 0]
  Delay : xbsIndex_r3/Delay  latency=1  reg_retiming=off  explicit_period=off  period=1  en=off  accept_only_valid=off  init_zero=on  dbl_ovrd=off  show_param=off
      settings: xl_area=[0, 0, 0, 0, 0, 0, 0]
  Logical1 : xbsIndex_r3/Logical  logical_function=OR  inputs=2  precision=Full  arith_type=Unsigned  n_bits=8  bin_pt=2  align_bp=on  latency=1  explicit_period=on  period=1  en=off  dbl_ovrd=off  show_param=off
      settings: xl_area=[0, 0, 0, 0, 0, 0, 0]
  Mux : xbsIndex_r3/Mux  inputs=2  precision=Full  arith_type="Signed  (2's comp)"  n_bits=8  bin_pt=2  quantization=Truncate  overflow=Wrap  latency=1  explicit_period=off  period=1  en=off  dbl_ovrd=off  show_param=off  mux_type=off  use_rpm=off  gen_core=on
      settings: xl_area=[0, 0, 0, 0, 0, 0, 0]
  Mux1 : xbsIndex_r3/Mux  inputs=2  precision=Full  arith_type="Signed  (2's comp)"  n_bits=8  bin_pt=2  quantization=Truncate  overflow=Wrap  latency=1  explicit_period=off  period=1  en=off  dbl_ovrd=off  show_param=off  mux_type=off  use_rpm=off  gen_core=on
      settings: xl_area=[0, 0, 0, 0, 0, 0, 0]
  Slice : xbsIndex_r3/Slice  Orientation=up  mode=Lower Bit Location + Width  nbits=1  bit1=-(FFTStage - 1)  base1=MSB of Input  bit0=FFTStage - 1  base0=LSB of Input  boolean_output=on  explicit_period=off  period=1  dbl_ovrd=off
  Slice1 : xbsIndex_r3/Slice  mode=Upper Bit Location + Width  nbits=1  bit1=0  base1=MSB of Input  bit0=0  base0=LSB of Input  boolean_output=off  explicit_period=off  period=1  dbl_ovrd=off
  butterfly : Subsystem
  delay_b : Subsystem  BlockChoice=delay_slr
      link override delay_bram: DelayLen=2^(FFTSize-FFTStage)  bram_latency=bram_latency
      link override delay_bram/Constant2: equ=P=C
      link override delay_slr: DelayLen=2^(FFTSize-FFTStage)
      settings: AttributesFormatString=%<BlockChoice>  TemplateBlock=delay_lib/delay  MemberBlocks=delay_bram,delay_slr
  delay_f : Subsystem  BlockChoice=delay_slr
      link override delay_bram: DelayLen=2^(FFTSize-FFTStage)  bram_latency=bram_latency
      link override delay_bram/Constant2: equ=P=C
      link override delay_slr: DelayLen=2^(FFTSize-FFTStage)
      settings: AttributesFormatString=%<BlockChoice>  TemplateBlock=delay_lib/delay  MemberBlocks=delay_bram,delay_slr
  sync_delay_x : fft_library/sync_delay  DelayLen=2^(FFTSize - FFTStage)
      link override Constant: equ=P=C
      link override Constant1: equ=P=C
      link override Constant2: equ=P=C
      link override Constant3: equ=P=C
  out1 : Outport
  out2 : Outport  Port=2
  of : Outport  Port=3
  sync_out : Outport  Port=4
  wires:
  shift/1 -> Slice/1
  of_in/1 -> Logical1/2
  Logical1/1 -> of/1
  Delay/1 -> sync_delay_x/1
  sync/1 -> Counter/1, Delay/1
  Counter/1 -> Slice1/1
  Mux/1 -> butterfly/2(b)
  Mux1/1 -> delay_b/1(In1)
  delay_f/1(Out1) -> Mux1/3, Mux/2
  in1/1 -> Mux/3, Mux1/2
  Slice1/1 -> Mux/1, Mux1/1
  in2/1 -> delay_f/1(In1)
  delay_b/1(Out1) -> butterfly/1(a)
  sync_delay_x/1 -> butterfly/3(sync)
  Slice/1 -> butterfly/4(shift)
  butterfly/3(of) -> Logical1/1
  butterfly/2(a-bw) -> out2/1
  butterfly/1(a+bw) -> out1/1
  butterfly/4(sync_out) -> sync_out/1

== system fft_library/fft_unscrambler ==
  sync : Inport  Port=1  LatchInput=off
  In1 : Inport  Port=2  LatchInput=off
  In2 : Inport  Port=3  LatchInput=off
  const : xbsIndex_r3/Constant  const=1  equ=P=C  arith_type=Boolean  n_bits=1  bin_pt=0  opselect=C  inp2=PCIN>>17  opr=+  inp1=P  carry=CIN  iostate=0  explicit_period=on  period=1  dbl_ovrd=off
  reorder : reorder_library/reorder  map=[0 2 4 6 8 10 12 14 16 18 20 22 24 26 28 30 1 3 5 7 9 11 13 15 17 19 21 23 25 27 29 31]  n_inputs=2^n_inputs  bram_latency=bram_latency  map_latency=1
  square_transposer : reorder_library/square_transposer  n_inputs=n_inputs
  sync_out : Outport
  Out1 : Outport  Port=2
  Out2 : Outport  Port=3
  wires:
  sync/1 -> square_transposer/1
  square_transposer/1 -> reorder/1
  reorder/1 -> sync_out/1
  const/1 -> reorder/2
  In1/1 -> square_transposer/2
  square_transposer/2 -> reorder/3
  reorder/3 -> Out1/1
  In2/1 -> square_transposer/3
  square_transposer/3 -> reorder/4
  reorder/4 -> Out2/1

== system fft_library/mirror_spectrum ==
  sync : Inport  Port=1  LatchInput=off
  din : Inport  Port=2  LatchInput=off
  reo_in : Inport  Port=3  LatchInput=off
  Constant3 : xbsIndex_r3/Constant  const=2^(FFTSize - 1)  equ=P=C  arith_type=Unsigned  n_bits=FFTSize  bin_pt=0  opselect=C  inp2=PCIN>>17  opr=+  inp1=P  carry=CIN  iostate=0  explicit_period=on  period=1  dbl_ovrd=off
  Counter : xbsIndex_r3/Counter  cnt_type=Free Running  n_bits=FFTSize  bin_pt=0  arith_type=Unsigned  start_count=0  cnt_to=Inf  cnt_by_val=1  operation=Up  explicit_period=off  period=1  load_pin=off  rst=on  en=off  dbl_ovrd=off  show_param=off  use_rpm=on  gen_core=off
      settings: xl_area=[0, 0, 0, 0, 0, 0, 0]
  Delay1 : xbsIndex_r3/Delay  latency=reorder_latency - 2  reg_retiming=off  explicit_period=off  period=1  en=off  accept_only_valid=off  init_zero=on  dbl_ovrd=off  show_param=off
      settings: xl_area=[0, 0, 0, 0, 0, 0, 0]
  Delay2 : xbsIndex_r3/Delay  latency=2  reg_retiming=off  explicit_period=off  period=1  en=off  accept_only_valid=off  init_zero=on  dbl_ovrd=off  show_param=off
      settings: xl_area=[0, 0, 0, 0, 0, 0, 0]
  Delay3 : xbsIndex_r3/Delay  latency=reorder_latency - 1  reg_retiming=off  explicit_period=off  period=1  en=off  accept_only_valid=off  init_zero=on  dbl_ovrd=off  show_param=off
      settings: xl_area=[0, 0, 0, 0, 0, 0, 0]
  Mux : xbsIndex_r3/Mux  inputs=2  precision=Full  arith_type="Signed  (2's comp)"  n_bits=8  bin_pt=2  quantization=Truncate  overflow=Wrap  latency=1  explicit_period=off  period=1  en=off  dbl_ovrd=off  show_param=off  mux_type=off  use_rpm=off  gen_core=off
      settings: xl_area=[0, 0, 0, 0, 0, 0, 0]
  Negate : xbsIndex_r3/Negate  precision=User Defined  arith_type=Unsigned  n_bits=n_bits  bin_pt=n_bits - 1  quantization=Truncate  overflow=Wrap  latency=0  explicit_period=off  period=1  en=off  dbl_ovrd=off  use_core=on  show_param=off  use_rpm=on  gen_core=off
      settings: xl_area=[0, 0, 0, 0, 0, 0, 0]
  Relational : xbsIndex_r3/Relational  mode=a>b  latency=1  explicit_period=off  period=1  en=off  dbl_ovrd=off  show_param=off
      settings: xl_area=[0, 0, 0, 0, 0, 0, 0]
  c_to_ri : fft_library/c_to_ri  BitWidth=n_bits
  ri_to_c : fft_library/ri_to_c  likes_cookies=off
  sync_out : Outport
  dout : Outport  Port=2
  wires:
  sync/1 -> Delay1/1
  Counter/1 -> Relational/1
  Constant3/1 -> Relational/2
  Relational/1 -> Mux/1
  din/1 -> Delay3/1
  Delay3/1 -> Mux/2
  Delay1/1 -> Counter/1, Delay2/1
  Mux/1 -> dout/1
  Delay2/1 -> sync_out/1
  reo_in/1 -> c_to_ri/1
  c_to_ri/1 -> ri_to_c/1
  ri_to_c/1 -> Mux/3
  c_to_ri/2 -> Negate/1
  Negate/1 -> ri_to_c/2
